simulink model "beamng_simulink_interface_demos"  (R2022b)
settings: Solver=FixedStepAuto  StartTime=0.0  StopTime=20  FixedStep=0.005  RelTol=1e-3
undefined symbols (not defined in the file): demo, mode
libraries: simulink x11, slpidlib x4, BeamNG_interface x1
settings Model: Creator=matti  LastModifiedBy=matti
settings SolverCC: AlgebraicLoopSolver=TrustRegion
settings DebuggingCC: ArithmeticOperatorsInVariantConditions=warning
settings SFSimCC: CustomCodeUndefinedFunction=UseInterfaceOnly

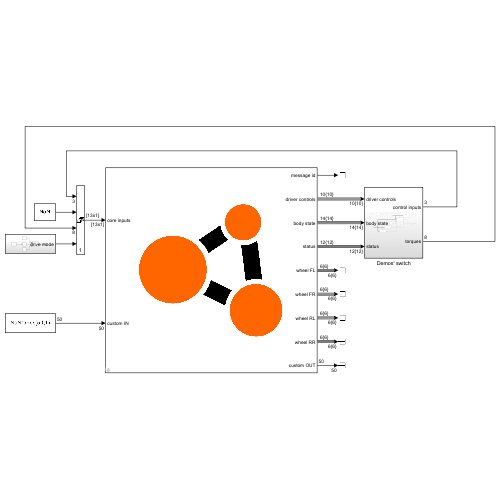
[thumbnail: Simulink's stored preview of the top-level diagram]
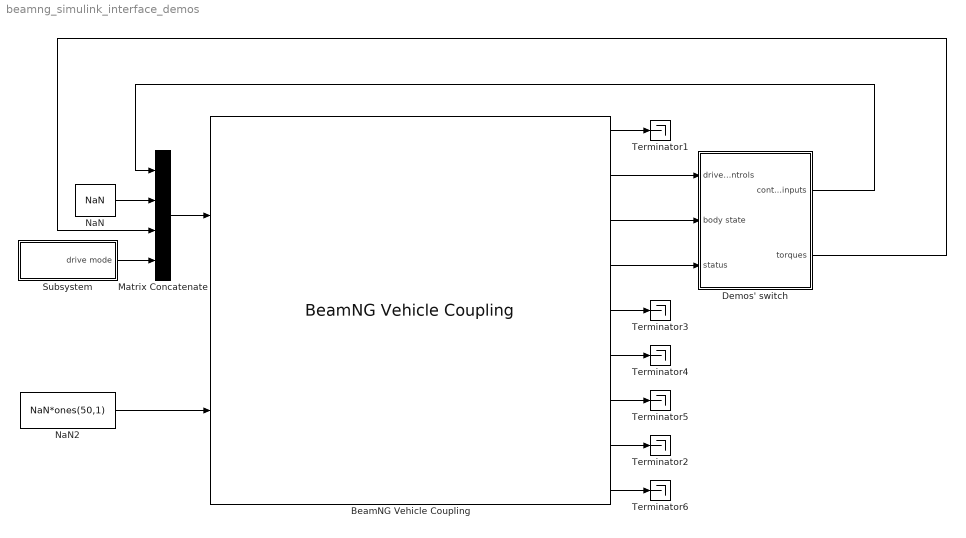
== system beamng_simulink_interface_demos ==
  BeamNG Vehicle Coupling : BeamNG_interface/BeamNG Vehicle Coupling
      settings: SourceProductName=BeamNG
  Demos' switch : Subsystem
  Matrix Concatenate : Concatenate  NumInputs=4  Mode=Multidimensional array
  NaN : Constant  Value=NaN  OutDataTypeStr=Inherit: Inherit via back propagation
  NaN2 : Constant  Value=NaN*ones(50,1)  OutDataTypeStr=Inherit: Inherit via back propagation
  Subsystem : Subsystem
  Terminator{1..6} (6 alike) : Terminator
  wires:
  Matrix Concatenate/1 -> BeamNG Vehicle Coupling/1
  NaN2/1 -> BeamNG Vehicle Coupling/2
  NaN/1 -> Matrix Concatenate/2
  BeamNG Vehicle Coupling/5 -> Terminator3/1
  BeamNG Vehicle Coupling/6 -> Terminator4/1
  BeamNG Vehicle Coupling/7 -> Terminator5/1
  BeamNG Vehicle Coupling/9 -> Terminator6/1
  Demos' switch/1(control inputs) -> Matrix Concatenate/1
  Demos' switch/2(torques) -> Matrix Concatenate/3
  Subsystem/1(drive mode) -> Matrix Concatenate/4
  BeamNG Vehicle Coupling/8 -> Terminator2/1
  BeamNG Vehicle Coupling/4 -> Demos' switch/3(status)
  BeamNG Vehicle Coupling/3 -> Demos' switch/2(body state)
  BeamNG Vehicle Coupling/2 -> Demos' switch/1(driver controls)
  BeamNG Vehicle Coupling/1 -> Terminator1/1

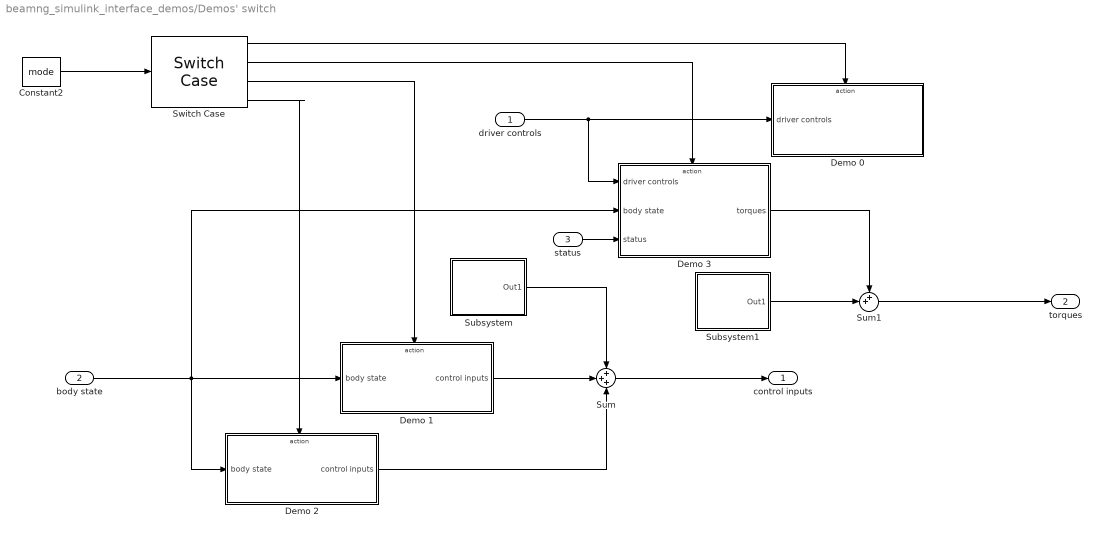
== system beamng_simulink_interface_demos/Demos' switch ==
  driver controls : Inport
  body state : Inport  Port=2
  status : Inport  Port=3
  Constant2 : Constant  Value=mode
  Demo 0 : Subsystem  TreatAsAtomicUnit=on
  Demo 1 : Subsystem  TreatAsAtomicUnit=on
  Demo 2 : Subsystem  TreatAsAtomicUnit=on
  Demo 3 : Subsystem  TreatAsAtomicUnit=on
  Subsystem : Subsystem
  Subsystem1 : Subsystem
  Sum : Sum  Inputs=+++
  Sum1 : Sum  Inputs=++|
  Switch Case : SwitchCase  CaseConditions={0, 3, 1, 2}  ShowDefaultCase=off
  control inputs : Outport
  torques : Outport  Port=2
  wires:
  Constant2/1 -> Switch Case/1
  Switch Case/1 -> Demo 0/Action
  Demo 2/1(control inputs) -> Sum/3
  driver controls/1 -> Demo 0/1(driver controls), Demo 3/1(driver controls)
  body state/1 -> Demo 3/2(body state), Demo 2/1(body state), Demo 1/1(body state)
  Sum/1 -> control inputs/1
  Subsystem/1(Out1) -> Sum/1
  Switch Case/4 -> Demo 2/Action
  Switch Case/3 -> Demo 1/Action
  Demo 1/1(control inputs) -> Sum/2
  Switch Case/2 -> Demo 3/Action
  Subsystem1/1(Out1) -> Sum1/2
  Demo 3/1(torques) -> Sum1/1
  Sum1/1 -> torques/1
  status/1 -> Demo 3/3(status)

== system beamng_simulink_interface_demos/Subsystem ==
  Compare To Constant : simulink/Logic and Bit Operations/Compare To Constant  relop===  const=3  OutDataTypeStr=boolean
  Constant : Constant  Value=mode
  Constant1 : Constant  Value=0
  Constant2 : Constant
  Switch : Switch  Criteria=u2 > Threshold  SaturateOnIntegerOverflow=off  InputSameDT=off
  drive mode : Outport
  wires:
  Constant/1 -> Compare To Constant/1
  Compare To Constant/1 -> Switch/2
  Constant1/1 -> Switch/3
  Constant2/1 -> Switch/1
  Switch/1 -> drive mode/1

== system beamng_simulink_interface_demos/Demos' switch/Demo 0 ==
  driver controls : Inport
  Action Port : ActionPort  ActionPortLabel=case [ 0 ]:
  Bus Selector : BusSelector  OutputSignals=throttle,brake,steering
  Scope : Scope  NumInputPorts=3
  To Workspace : ToWorkspace  VariableName=throttle0  SaveFormat=Timeseries  SampleTime=-1
  To Workspace1 : ToWorkspace  VariableName=brake0  SaveFormat=Timeseries  SampleTime=-1
  To Workspace2 : ToWorkspace  VariableName=steering0  SaveFormat=Timeseries  SampleTime=-1
  wires:
  driver controls/1 -> Bus Selector/1
  Bus Selector/1 -> To Workspace/1, Scope/1  "<throttle>"
  Bus Selector/2 -> To Workspace1/1, Scope/2  "<brake>"
  Bus Selector/3 -> To Workspace2/1, Scope/3  "<steering>"

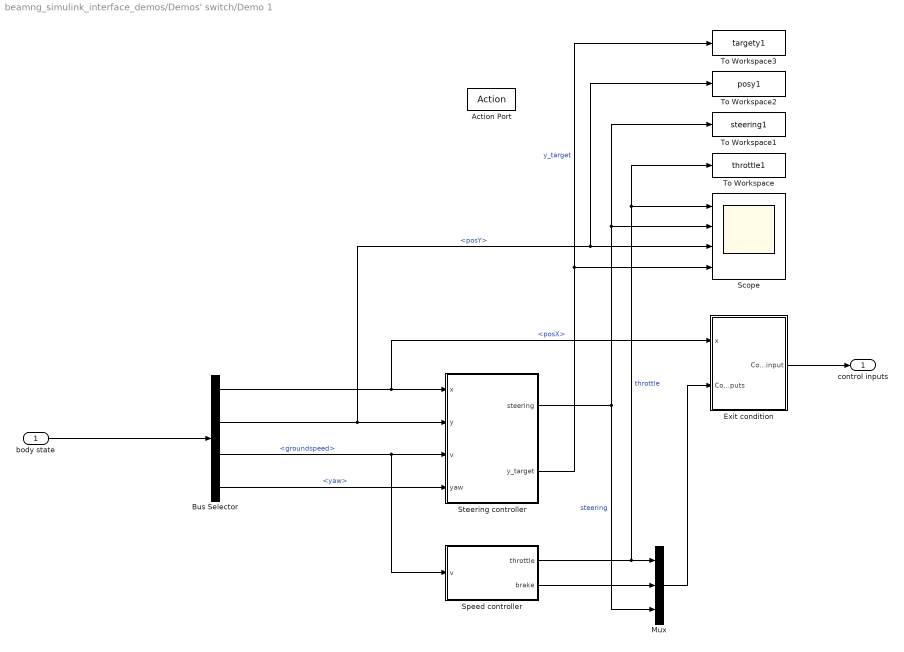
== system beamng_simulink_interface_demos/Demos' switch/Demo 1 ==
  body state : Inport
  Action Port : ActionPort  ActionPortLabel=case [ 1 ]:
  Bus Selector : BusSelector  OutputSignals=posX,posY,groundspeed,yaw
  Exit condition : Subsystem
  Mux : Mux  Inputs=3
  Scope : Scope  NumInputPorts=4
  Speed controller : Subsystem
  Steering controller : Subsystem
  To Workspace : ToWorkspace  VariableName=throttle1  SaveFormat=Timeseries  SampleTime=-1
  To Workspace1 : ToWorkspace  VariableName=steering1  SaveFormat=Timeseries  SampleTime=-1
  To Workspace2 : ToWorkspace  VariableName=posy1  SaveFormat=Timeseries  SampleTime=-1
  To Workspace3 : ToWorkspace  VariableName=targety1  SaveFormat=Timeseries  SampleTime=-1
  control inputs : Outport
  wires:
  Bus Selector/4 -> Steering controller/4(yaw)  "<yaw>"
  Speed controller/2(brake) -> Mux/2
  Exit condition/1(Control input) -> control inputs/1
  Mux/1 -> Exit condition/2(Control inputs)
  Speed controller/1(throttle) -> Mux/1, To Workspace/1, Scope/1  "throttle"
  body state/1 -> Bus Selector/1
  Bus Selector/2 -> Steering controller/2(y), To Workspace2/1, Scope/3  "<posY>"
  Bus Selector/1 -> Exit condition/1(x), Steering controller/1(x)  "<posX>"
  Steering controller/2(y_target) -> To Workspace3/1, Scope/4  "y_target"
  Bus Selector/3 -> Speed controller/1(v), Steering controller/3(v)  "<groundspeed>"
  Steering controller/1(steering) -> Mux/3, To Workspace1/1, Scope/2  "steering"

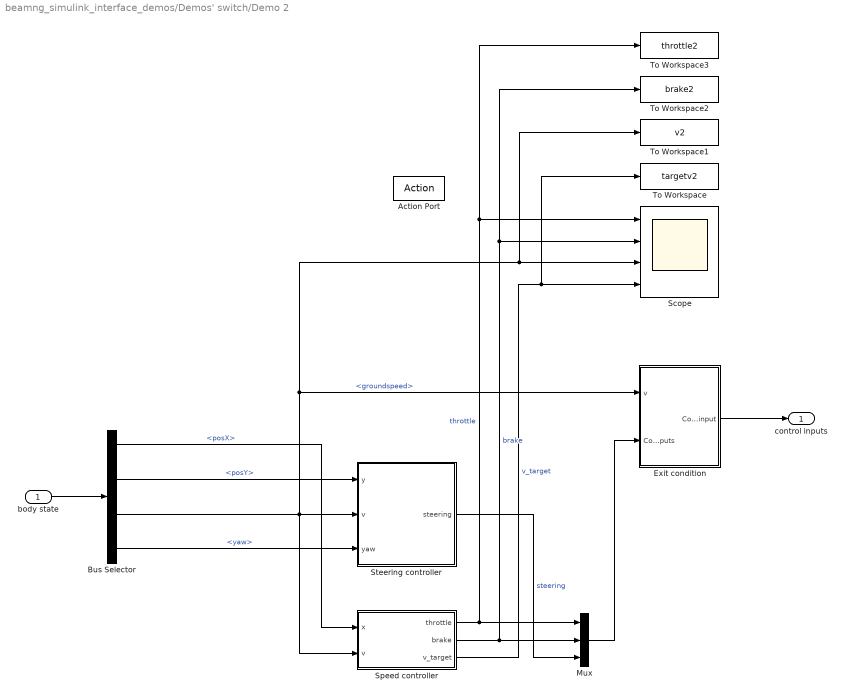
== system beamng_simulink_interface_demos/Demos' switch/Demo 2 ==
  body state : Inport
  Action Port : ActionPort  ActionPortLabel=case [ 2 ]:
  Bus Selector : BusSelector  OutputSignals=posX,posY,groundspeed,yaw
  Exit condition : Subsystem
  Mux : Mux  Inputs=3
  Scope : Scope  NumInputPorts=4
  Speed controller : Subsystem
  Steering controller : Subsystem
  To Workspace : ToWorkspace  VariableName=targetv2  SaveFormat=Timeseries  SampleTime=-1
  To Workspace1 : ToWorkspace  VariableName=v2  SaveFormat=Timeseries  SampleTime=-1
  To Workspace2 : ToWorkspace  VariableName=brake2  SaveFormat=Timeseries  SampleTime=-1
  To Workspace3 : ToWorkspace  VariableName=throttle2  SaveFormat=Timeseries  SampleTime=-1
  control inputs : Outport
  wires:
  Speed controller/3(v_target) -> To Workspace/1, Scope/4  "v_target"
  Exit condition/1(Control input) -> control inputs/1
  Speed controller/2(brake) -> Mux/2, To Workspace2/1, Scope/2  "brake"
  Steering controller/1(steering) -> Mux/3  "steering"
  Speed controller/1(throttle) -> Mux/1, To Workspace3/1, Scope/1  "throttle"
  body state/1 -> Bus Selector/1
  Bus Selector/4 -> Steering controller/3(yaw)  "<yaw>"
  Mux/1 -> Exit condition/2(Control inputs)
  Bus Selector/3 -> Speed controller/2(v), To Workspace1/1, Scope/3, Exit condition/1(v), Steering controller/2(v)  "<groundspeed>"
  Bus Selector/2 -> Steering controller/1(y)  "<posY>"
  Bus Selector/1 -> Speed controller/1(x)  "<posX>"

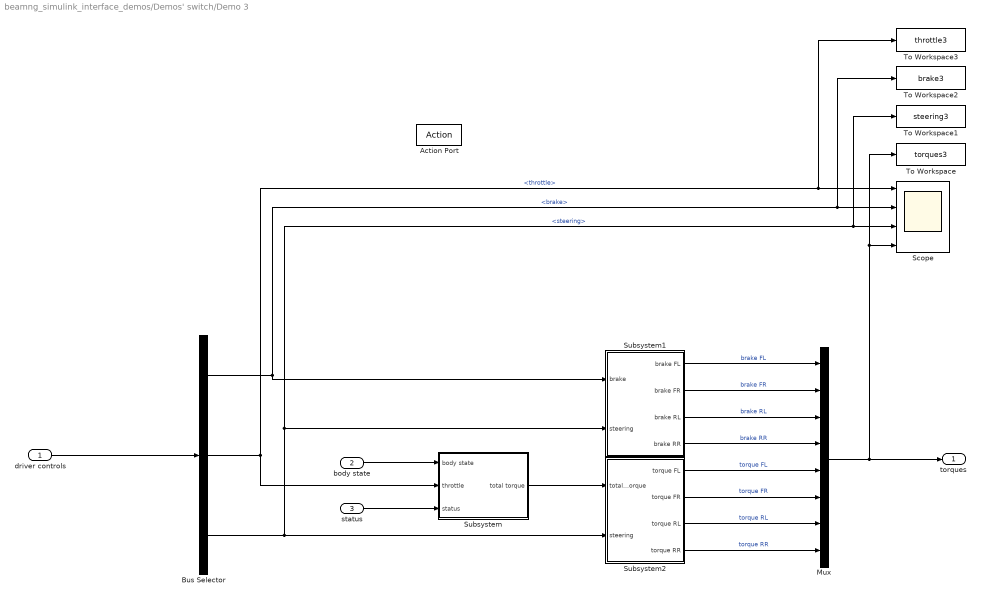
== system beamng_simulink_interface_demos/Demos' switch/Demo 3 ==
  driver controls : Inport
  body state : Inport  Port=2
  status : Inport  Port=3
  Action Port : ActionPort  ActionPortLabel=case [ 3 ]:
  Bus Selector : BusSelector  OutputSignals=brake,throttle,steering
  Mux : Mux  Inputs=8
  Scope : Scope  NumInputPorts=4
  Subsystem : Subsystem
  Subsystem1 : Subsystem
  Subsystem2 : Subsystem
  To Workspace : ToWorkspace  VariableName=torques3  SaveFormat=Timeseries  SampleTime=-1
  To Workspace1 : ToWorkspace  VariableName=steering3  SaveFormat=Timeseries  SampleTime=-1
  To Workspace2 : ToWorkspace  VariableName=brake3  SaveFormat=Timeseries  SampleTime=-1
  To Workspace3 : ToWorkspace  VariableName=throttle3  SaveFormat=Timeseries  SampleTime=-1
  torques : Outport
  wires:
  driver controls/1 -> Bus Selector/1
  Bus Selector/1 -> Subsystem1/1(brake), To Workspace2/1, Scope/2  "<brake>"
  Bus Selector/2 -> Subsystem/2(throttle), To Workspace3/1, Scope/1  "<throttle>"
  Bus Selector/3 -> Subsystem1/2(steering), To Workspace1/1, Scope/3, Subsystem2/2(steering)  "<steering>"
  body state/1 -> Subsystem/1(body state)
  status/1 -> Subsystem/3(status)
  Subsystem1/1(brake FL) -> Mux/1  "brake FL"
  Subsystem1/2(brake FR) -> Mux/2  "brake FR"
  Subsystem1/3(brake RL) -> Mux/3  "brake RL"
  Subsystem1/4(brake RR) -> Mux/4  "brake RR"
  Subsystem/1(total torque) -> Subsystem2/1(total torque)
  Subsystem2/1(torque FL) -> Mux/5  "torque FL"
  Subsystem2/2(torque FR) -> Mux/6  "torque FR"
  Subsystem2/3(torque RL) -> Mux/7  "torque RL"
  Subsystem2/4(torque RR) -> Mux/8  "torque RR"
  Mux/1 -> torques/1, To Workspace/1, Scope/4

== system beamng_simulink_interface_demos/Demos' switch/Subsystem ==
  Compare To Constant : simulink/Logic and Bit Operations/Compare To Constant  relop===  const=0  OutDataTypeStr=boolean
  Compare To Constant1 : simulink/Logic and Bit Operations/Compare To Constant  relop===  const=3  OutDataTypeStr=boolean
  Constant : Constant  Value=mode
  NaN : Constant  Value=NaN*ones(3,1)  OutDataTypeStr=Inherit: Inherit via back propagation
  NaN2 : Constant  Value=zeros(3,1)  OutDataTypeStr=Inherit: Inherit via back propagation
  OR : Logic  Operator=OR  IconShape=distinctive  AllPortsSameDT=off  OutDataTypeStr=boolean
  Switch : Switch  Criteria=u2 > Threshold  SaturateOnIntegerOverflow=off  InputSameDT=off
  Out1 : Outport
  wires:
  Constant/1 -> Compare To Constant1/1, Compare To Constant/1
  NaN/1 -> Switch/1
  Compare To Constant/1 -> OR/1
  OR/1 -> Switch/2
  NaN2/1 -> Switch/3
  Switch/1 -> Out1/1
  Compare To Constant1/1 -> OR/2

== system beamng_simulink_interface_demos/Demos' switch/Subsystem1 ==
  Compare To Constant1 : simulink/Logic and Bit Operations/Compare To Constant  relop===  const=3  OutDataTypeStr=boolean
  Constant : Constant  Value=mode
  NaN : Constant  Value=NaN*ones(8,1)  OutDataTypeStr=Inherit: Inherit via back propagation
  NaN2 : Constant  Value=zeros(8,1)  OutDataTypeStr=Inherit: Inherit via back propagation
  Switch : Switch  Criteria=u2 > Threshold  SaturateOnIntegerOverflow=off  InputSameDT=off
  Out1 : Outport
  wires:
  Switch/1 -> Out1/1
  Compare To Constant1/1 -> Switch/2
  Constant/1 -> Compare To Constant1/1
  NaN2/1 -> Switch/1
  NaN/1 -> Switch/3

== system beamng_simulink_interface_demos/Demos' switch/Demo 1/Exit condition ==
  x : Inport
  Control inputs : Inport  Port=2
  Constant3 : Constant
  Stop Simulation : Stop
  Switch1 : Switch  Threshold=demo(1).x4  SaturateOnIntegerOverflow=off  InputSameDT=off
  Switch2 : Switch  Criteria=u2 > Threshold  Threshold=demo(1).x4  SaturateOnIntegerOverflow=off  InputSameDT=off
  Zero : Constant  Value=0  OutDataTypeStr=Inherit: Inherit via back propagation
  Zero1 : Constant  Value=zeros(3,1)  OutDataTypeStr=Inherit: Inherit via back propagation
  Control input : Outport
  wires:
  Zero/1 -> Switch2/3
  x/1 -> Switch1/2, Switch2/2
  Switch2/1 -> Stop Simulation/1
  Constant3/1 -> Switch2/1
  Control inputs/1 -> Switch1/3
  Switch1/1 -> Control input/1
  Zero1/1 -> Switch1/1

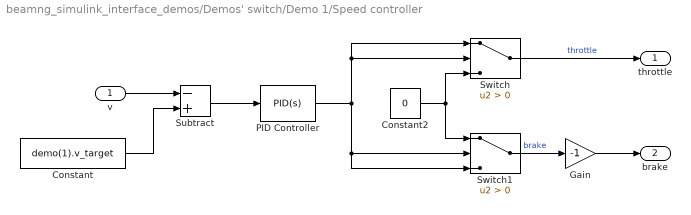
== system beamng_simulink_interface_demos/Demos' switch/Demo 1/Speed controller ==
  v : Inport
  Constant : Constant  Value=demo(1).v_target
  Constant2 : Constant  Value=0
  Gain : Gain  Gain=-1
  PID Controller : slpidlib/PID Controller  Controller=PID  Form=Parallel  TimeDomain=Continuous-time  UseExternalTs=off  SampleTime=-1  IntegratorMethod=Forward Euler  FilterMethod=Forward Euler  ControllerParametersSource=internal  P=0.1  I=0.01  UseKiTs=off  D=0  N=100  UseFilter=on  TunerSelectOption=Transfer Function Based (PID Tuner App)  InitialConditionSource=internal  InitialConditionForIntegrator=0  InitialConditionForFilter=0  DifferentiatorICPrevScaledInput=0  ExternalReset=none  TrackingMode=off  Kt=1  LimitOutput=on  SatLimitsSource=internal  UpperSaturationLimit=1  LowerSaturationLimit=-1  LinearizeAsGain=on  AntiWindupMode=none  Kb=1  LimitIntegrator=off  UpperIntegratorSaturationLimit=inf  LowerIntegratorSaturationLimit=-inf  POutMin=[]  POutMax=[]  IOutMin=[]  IOutMax=[]  DOutMin=[]  DOutMax=[]  NOutMin=[]  NOutMax=[]  SumOutMin=[]  SumOutMax=[]  SaturationOutMin=[]  SaturationOutMax=[]  PParamMin=[]  PParamMax=[]  IParamMin=[]  IParamMax=[]  DParamMin=[]  DParamMax=[]  NParamMin=[]  NParamMax=[]  KbParamMin=[]  KbParamMax=[]  KtParamMin=[]  KtParamMax=[]  KbOutMin=[]  KbOutMax=[]  KtOutMin=[]  KtOutMax=[]  IntegratorOutMin=[]  IntegratorOutMax=[]  FilterOutMin=[]  FilterOutMax=[]  SumI1OutMin=[]  SumI1OutMax=[]  SumI2OutMin=[]  SumI2OutMax=[]  SumI3OutMin=[]  SumI3OutMax=[]  SumI4OutMin=[]  SumI4OutMax=[]  SumDOutMin=[]  SumDOutMax=[]  DifferentiatorOutMin=[]  DifferentiatorOutMax=[]  FilterDiffOutCoefMin=[]  FilterDiffOutCoefMax=[]  ReciprocalOutMin=[]  ReciprocalOutMax=[]  SumDenOutMin=[]  SumDenOutMax=[]  SumNumOutMin=[]  SumNumOutMax=[]  DivideOutMin=[]  DivideOutMax=[]  UdiffTsProdOutMin=[]  UdiffTsProdOutMax=[]  NTsProdOutMin=[]  NTsProdOutMax=[]  UintegralTsProdOutMin=[]  UintegralTsProdOutMax=[]  UngainTsProdOutMin=[]  UngainTsProdOutMax=[]  ClampingZeroOutDataTypeStr=Inherit: Inherit via back propagation  ClampingZeroOutMin=[]  ClampingZeroOutMax=[]  FilterDenConstantOutDataTypeStr=Inherit: Inherit via back propagation  FilterDenConstantOutMin=[]  FilterDenConstantOutMax=[]  PCopyOutDataTypeStr=Inherit: Inherit via back propagation  PCopyOutMin=[]  PCopyOutMax=[]  NCopyOutDataTypeStr=Inherit: Inherit via back propagation  NCopyOutMin=[]  NCopyOutMax=[]  IntegratorContinuousStateAttributes=''  IntegratorStateMustResolveToSignalObject=off  IntegratorRTWStateStorageClass=Auto  FilterContinuousStateAttributes=''  FilterStateMustResolveToSignalObject=off  FilterRTWStateStorageClass=Auto  ParallelPVariant=InternalParameters  IdealPVariant=Disabled  IVariant=InternalParameters  DVariant=InternalParameters  IntegratorVariant=Continuous  SatVariant=Enabled  AWVariant=Passthrough  PCopyVariant=Disabled  TRVariant=Disabled  FdbkBlocksVariant=Forward  IdealPFdbkVariant=Disabled  SatFdbkVariant=Disabled  DerivativeFilterVariant=ContFilter  NVariant=InternalParameters  NCopyVariant=Disabled  FilterICVariant=InternalICsFilter  IntegratorICVariant=InternalICs  ExternalResetVariant=Disabled  TRSumVariant=Passthrough  SumFdbkVariant=Disabled  SumVariant=Sum_PID  TsampFilterVariant=InternalTs  TsampNgainVariant=Passthrough  TsampIntegralVariant=Passthrough  ExternalSaturationOutDataTypeStr=Inherit: Same as second input
  Subtract : Sum  Inputs=-+
  Switch : Switch  Criteria=u2 > Threshold  SaturateOnIntegerOverflow=off  InputSameDT=off
  Switch1 : Switch  Criteria=u2 > Threshold  SaturateOnIntegerOverflow=off  InputSameDT=off
  throttle : Outport
  brake : Outport  Port=2
  wires:
  PID Controller/1 -> Switch/2, Switch/1, Switch1/2, Switch1/3
  v/1 -> Subtract/1
  Constant2/1 -> Switch/3, Switch1/1
  Switch1/1 -> Gain/1  "brake"
  Constant/1 -> Subtract/2
  Subtract/1 -> PID Controller/1
  Switch/1 -> throttle/1  "throttle"
  Gain/1 -> brake/1

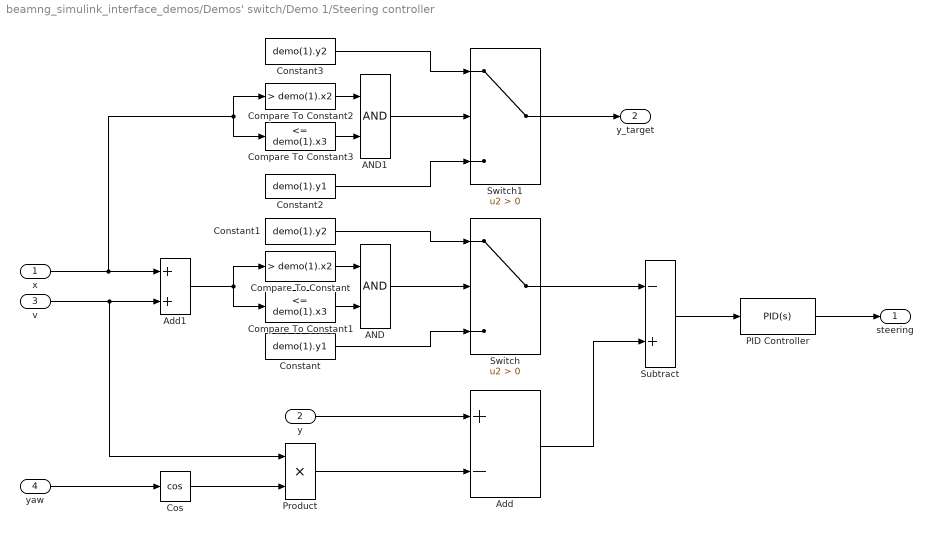
== system beamng_simulink_interface_demos/Demos' switch/Demo 1/Steering controller ==
  x : Inport
  y : Inport  Port=2
  v : Inport  Port=3
  yaw : Inport  Port=4
  AND : Logic  IconShape=distinctive  AllPortsSameDT=off  OutDataTypeStr=boolean
  AND1 : Logic  IconShape=distinctive  AllPortsSameDT=off  OutDataTypeStr=boolean
  Add : Sum  Inputs=+-
  Add1 : Sum
  Compare To Constant : simulink/Logic and Bit Operations/Compare To Constant  relop=>  const=demo(1).x2  OutDataTypeStr=boolean
  Compare To Constant1 : simulink/Logic and Bit Operations/Compare To Constant  relop=<=  const=demo(1).x3  OutDataTypeStr=boolean
  Compare To Constant2 : simulink/Logic and Bit Operations/Compare To Constant  relop=>  const=demo(1).x2  OutDataTypeStr=boolean
  Compare To Constant3 : simulink/Logic and Bit Operations/Compare To Constant  relop=<=  const=demo(1).x3  OutDataTypeStr=boolean
  Constant : Constant  Value=demo(1).y1
  Constant1 : Constant  Value=demo(1).y2
  Constant2 : Constant  Value=demo(1).y1
  Constant3 : Constant  Value=demo(1).y2
  Cos : Trigonometry  Operator=cos
  PID Controller : slpidlib/PID Controller  Controller=PID  Form=Parallel  TimeDomain=Continuous-time  UseExternalTs=off  SampleTime=-1  IntegratorMethod=Forward Euler  FilterMethod=Forward Euler  ControllerParametersSource=internal  P=0.05  I=0  UseKiTs=off  D=0  N=100  UseFilter=on  TunerSelectOption=Transfer Function Based (PID Tuner App)  InitialConditionSource=internal  InitialConditionForIntegrator=0  InitialConditionForFilter=0  DifferentiatorICPrevScaledInput=0  ExternalReset=none  TrackingMode=off  Kt=1  LimitOutput=on  SatLimitsSource=internal  UpperSaturationLimit=1  LowerSaturationLimit=-1  LinearizeAsGain=on  AntiWindupMode=none  Kb=1  LimitIntegrator=off  UpperIntegratorSaturationLimit=inf  LowerIntegratorSaturationLimit=-inf  POutMin=[]  POutMax=[]  IOutMin=[]  IOutMax=[]  DOutMin=[]  DOutMax=[]  NOutMin=[]  NOutMax=[]  SumOutMin=[]  SumOutMax=[]  SaturationOutMin=[]  SaturationOutMax=[]  PParamMin=[]  PParamMax=[]  IParamMin=[]  IParamMax=[]  DParamMin=[]  DParamMax=[]  NParamMin=[]  NParamMax=[]  KbParamMin=[]  KbParamMax=[]  KtParamMin=[]  KtParamMax=[]  KbOutMin=[]  KbOutMax=[]  KtOutMin=[]  KtOutMax=[]  IntegratorOutMin=[]  IntegratorOutMax=[]  FilterOutMin=[]  FilterOutMax=[]  SumI1OutMin=[]  SumI1OutMax=[]  SumI2OutMin=[]  SumI2OutMax=[]  SumI3OutMin=[]  SumI3OutMax=[]  SumI4OutMin=[]  SumI4OutMax=[]  SumDOutMin=[]  SumDOutMax=[]  DifferentiatorOutMin=[]  DifferentiatorOutMax=[]  FilterDiffOutCoefMin=[]  FilterDiffOutCoefMax=[]  ReciprocalOutMin=[]  ReciprocalOutMax=[]  SumDenOutMin=[]  SumDenOutMax=[]  SumNumOutMin=[]  SumNumOutMax=[]  DivideOutMin=[]  DivideOutMax=[]  UdiffTsProdOutMin=[]  UdiffTsProdOutMax=[]  NTsProdOutMin=[]  NTsProdOutMax=[]  UintegralTsProdOutMin=[]  UintegralTsProdOutMax=[]  UngainTsProdOutMin=[]  UngainTsProdOutMax=[]  ClampingZeroOutDataTypeStr=Inherit: Inherit via back propagation  ClampingZeroOutMin=[]  ClampingZeroOutMax=[]  FilterDenConstantOutDataTypeStr=Inherit: Inherit via back propagation  FilterDenConstantOutMin=[]  FilterDenConstantOutMax=[]  PCopyOutDataTypeStr=Inherit: Inherit via back propagation  PCopyOutMin=[]  PCopyOutMax=[]  NCopyOutDataTypeStr=Inherit: Inherit via back propagation  NCopyOutMin=[]  NCopyOutMax=[]  IntegratorContinuousStateAttributes=''  IntegratorStateMustResolveToSignalObject=off  IntegratorRTWStateStorageClass=Auto  FilterContinuousStateAttributes=''  FilterStateMustResolveToSignalObject=off  FilterRTWStateStorageClass=Auto  ParallelPVariant=InternalParameters  IdealPVariant=Disabled  IVariant=InternalParameters  DVariant=InternalParameters  IntegratorVariant=Continuous  SatVariant=Enabled  AWVariant=Passthrough  PCopyVariant=Disabled  TRVariant=Disabled  FdbkBlocksVariant=Forward  IdealPFdbkVariant=Disabled  SatFdbkVariant=Disabled  DerivativeFilterVariant=ContFilter  NVariant=InternalParameters  NCopyVariant=Disabled  FilterICVariant=InternalICsFilter  IntegratorICVariant=InternalICs  ExternalResetVariant=Disabled  TRSumVariant=Passthrough  SumFdbkVariant=Disabled  SumVariant=Sum_PID  TsampFilterVariant=InternalTs  TsampNgainVariant=Passthrough  TsampIntegralVariant=Passthrough  ExternalSaturationOutDataTypeStr=Inherit: Same as second input
  Product : Product
  Subtract : Sum  Inputs=-+
  Switch : Switch  Criteria=u2 > Threshold  SaturateOnIntegerOverflow=off  InputSameDT=off
  Switch1 : Switch  Criteria=u2 > Threshold  SaturateOnIntegerOverflow=off  InputSameDT=off
  steering : Outport
  y_target : Outport  Port=2
  wires:
  v/1 -> Product/1, Add1/2
  Add1/1 -> Compare To Constant/1, Compare To Constant1/1
  Compare To Constant/1 -> AND/1
  Compare To Constant1/1 -> AND/2
  AND/1 -> Switch/2
  Constant1/1 -> Switch/1
  Constant/1 -> Switch/3
  Switch/1 -> Subtract/1
  PID Controller/1 -> steering/1
  Subtract/1 -> PID Controller/1
  yaw/1 -> Cos/1
  Cos/1 -> Product/2
  Product/1 -> Add/2
  y/1 -> Add/1
  Add/1 -> Subtract/2
  Switch1/1 -> y_target/1
  Constant2/1 -> Switch1/3
  Constant3/1 -> Switch1/1
  AND1/1 -> Switch1/2
  Compare To Constant3/1 -> AND1/2
  Compare To Constant2/1 -> AND1/1
  x/1 -> Compare To Constant2/1, Compare To Constant3/1, Add1/1

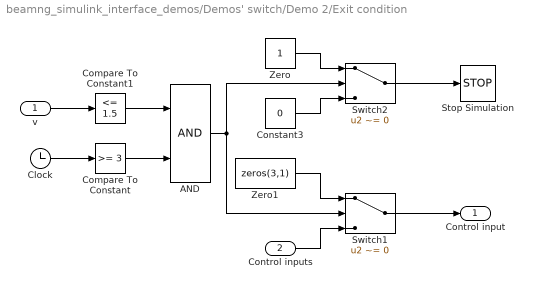
== system beamng_simulink_interface_demos/Demos' switch/Demo 2/Exit condition ==
  v : Inport
  Control inputs : Inport  Port=2
  AND : Logic  IconShape=distinctive  AllPortsSameDT=off  OutDataTypeStr=boolean
  Clock : Clock
  Compare To Constant : simulink/Logic and Bit Operations/Compare To Constant  relop=>=  const=3  OutDataTypeStr=boolean
  Compare To Constant1 : simulink/Logic and Bit Operations/Compare To Constant  relop=<=  const=1.5  OutDataTypeStr=boolean
  Constant3 : Constant  Value=0
  Stop Simulation : Stop
  Switch1 : Switch  Criteria=u2 ~= 0  SaturateOnIntegerOverflow=off  InputSameDT=off
  Switch2 : Switch  Criteria=u2 ~= 0  SaturateOnIntegerOverflow=off  InputSameDT=off
  Zero : Constant  OutDataTypeStr=Inherit: Inherit via back propagation
  Zero1 : Constant  Value=zeros(3,1)  OutDataTypeStr=Inherit: Inherit via back propagation
  Control input : Outport
  wires:
  Switch2/1 -> Stop Simulation/1
  Switch1/1 -> Control input/1
  Clock/1 -> Compare To Constant/1
  v/1 -> Compare To Constant1/1
  Compare To Constant1/1 -> AND/1
  Compare To Constant/1 -> AND/2
  Constant3/1 -> Switch2/3
  Zero/1 -> Switch2/1
  AND/1 -> Switch1/2, Switch2/2
  Zero1/1 -> Switch1/1
  Control inputs/1 -> Switch1/3

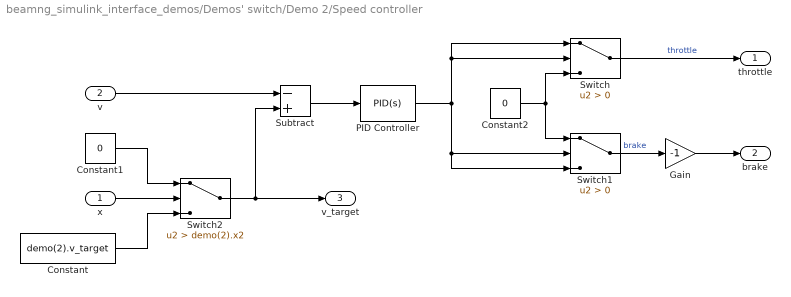
== system beamng_simulink_interface_demos/Demos' switch/Demo 2/Speed controller ==
  x : Inport
  v : Inport  Port=2
  Constant : Constant  Value=demo(2).v_target
  Constant1 : Constant  Value=0
  Constant2 : Constant  Value=0
  Gain : Gain  Gain=-1
  PID Controller : slpidlib/PID Controller  Controller=PID  Form=Parallel  TimeDomain=Continuous-time  UseExternalTs=off  SampleTime=-1  IntegratorMethod=Forward Euler  FilterMethod=Forward Euler  ControllerParametersSource=internal  P=0.3  I=0.001  UseKiTs=off  D=0  N=100  UseFilter=on  TunerSelectOption=Transfer Function Based (PID Tuner App)  InitialConditionSource=internal  InitialConditionForIntegrator=0  InitialConditionForFilter=0  DifferentiatorICPrevScaledInput=0  ExternalReset=none  TrackingMode=off  Kt=1  LimitOutput=on  SatLimitsSource=internal  UpperSaturationLimit=1  LowerSaturationLimit=-1  LinearizeAsGain=on  AntiWindupMode=none  Kb=1  LimitIntegrator=off  UpperIntegratorSaturationLimit=inf  LowerIntegratorSaturationLimit=-inf  POutMin=[]  POutMax=[]  IOutMin=[]  IOutMax=[]  DOutMin=[]  DOutMax=[]  NOutMin=[]  NOutMax=[]  SumOutMin=[]  SumOutMax=[]  SaturationOutMin=[]  SaturationOutMax=[]  PParamMin=[]  PParamMax=[]  IParamMin=[]  IParamMax=[]  DParamMin=[]  DParamMax=[]  NParamMin=[]  NParamMax=[]  KbParamMin=[]  KbParamMax=[]  KtParamMin=[]  KtParamMax=[]  KbOutMin=[]  KbOutMax=[]  KtOutMin=[]  KtOutMax=[]  IntegratorOutMin=[]  IntegratorOutMax=[]  FilterOutMin=[]  FilterOutMax=[]  SumI1OutMin=[]  SumI1OutMax=[]  SumI2OutMin=[]  SumI2OutMax=[]  SumI3OutMin=[]  SumI3OutMax=[]  SumI4OutMin=[]  SumI4OutMax=[]  SumDOutMin=[]  SumDOutMax=[]  DifferentiatorOutMin=[]  DifferentiatorOutMax=[]  FilterDiffOutCoefMin=[]  FilterDiffOutCoefMax=[]  ReciprocalOutMin=[]  ReciprocalOutMax=[]  SumDenOutMin=[]  SumDenOutMax=[]  SumNumOutMin=[]  SumNumOutMax=[]  DivideOutMin=[]  DivideOutMax=[]  UdiffTsProdOutMin=[]  UdiffTsProdOutMax=[]  NTsProdOutMin=[]  NTsProdOutMax=[]  UintegralTsProdOutMin=[]  UintegralTsProdOutMax=[]  UngainTsProdOutMin=[]  UngainTsProdOutMax=[]  ClampingZeroOutDataTypeStr=Inherit: Inherit via back propagation  ClampingZeroOutMin=[]  ClampingZeroOutMax=[]  FilterDenConstantOutDataTypeStr=Inherit: Inherit via back propagation  FilterDenConstantOutMin=[]  FilterDenConstantOutMax=[]  PCopyOutDataTypeStr=Inherit: Inherit via back propagation  PCopyOutMin=[]  PCopyOutMax=[]  NCopyOutDataTypeStr=Inherit: Inherit via back propagation  NCopyOutMin=[]  NCopyOutMax=[]  IntegratorContinuousStateAttributes=''  IntegratorStateMustResolveToSignalObject=off  IntegratorRTWStateStorageClass=Auto  FilterContinuousStateAttributes=''  FilterStateMustResolveToSignalObject=off  FilterRTWStateStorageClass=Auto  ParallelPVariant=InternalParameters  IdealPVariant=Disabled  IVariant=InternalParameters  DVariant=InternalParameters  IntegratorVariant=Continuous  SatVariant=Enabled  AWVariant=Passthrough  PCopyVariant=Disabled  TRVariant=Disabled  FdbkBlocksVariant=Forward  IdealPFdbkVariant=Disabled  SatFdbkVariant=Disabled  DerivativeFilterVariant=ContFilter  NVariant=InternalParameters  NCopyVariant=Disabled  FilterICVariant=InternalICsFilter  IntegratorICVariant=InternalICs  ExternalResetVariant=Disabled  TRSumVariant=Passthrough  SumFdbkVariant=Disabled  SumVariant=Sum_PID  TsampFilterVariant=InternalTs  TsampNgainVariant=Passthrough  TsampIntegralVariant=Passthrough  ExternalSaturationOutDataTypeStr=Inherit: Same as second input
  Subtract : Sum  Inputs=-+
  Switch : Switch  Criteria=u2 > Threshold  SaturateOnIntegerOverflow=off  InputSameDT=off
  Switch1 : Switch  Criteria=u2 > Threshold  SaturateOnIntegerOverflow=off  InputSameDT=off
  Switch2 : Switch  Criteria=u2 > Threshold  Threshold=demo(2).x2  SaturateOnIntegerOverflow=off  InputSameDT=off
  throttle : Outport
  brake : Outport  Port=2
  v_target : Outport  Port=3
  wires:
  PID Controller/1 -> Switch/2, Switch/1, Switch1/2, Switch1/3
  v/1 -> Subtract/1
  Constant2/1 -> Switch/3, Switch1/1
  Switch1/1 -> Gain/1  "brake"
  Subtract/1 -> PID Controller/1
  Switch/1 -> throttle/1  "throttle"
  x/1 -> Switch2/2
  Switch2/1 -> v_target/1, Subtract/2
  Gain/1 -> brake/1
  Constant1/1 -> Switch2/1
  Constant/1 -> Switch2/3

== system beamng_simulink_interface_demos/Demos' switch/Demo 2/Steering controller ==
  y : Inport
  v : Inport  Port=2
  yaw : Inport  Port=3
  Add : Sum  Inputs=+-
  Constant : Constant  Value=demo(2).y
  Cos : Trigonometry  Operator=cos
  PID Controller : slpidlib/PID Controller  Controller=PID  Form=Parallel  TimeDomain=Continuous-time  UseExternalTs=off  SampleTime=-1  IntegratorMethod=Forward Euler  FilterMethod=Forward Euler  ControllerParametersSource=internal  P=0.05  I=0  UseKiTs=off  D=0  N=100  UseFilter=on  TunerSelectOption=Transfer Function Based (PID Tuner App)  InitialConditionSource=internal  InitialConditionForIntegrator=0  InitialConditionForFilter=0  DifferentiatorICPrevScaledInput=0  ExternalReset=none  TrackingMode=off  Kt=1  LimitOutput=on  SatLimitsSource=internal  UpperSaturationLimit=1  LowerSaturationLimit=-1  LinearizeAsGain=on  AntiWindupMode=none  Kb=1  LimitIntegrator=off  UpperIntegratorSaturationLimit=inf  LowerIntegratorSaturationLimit=-inf  POutMin=[]  POutMax=[]  IOutMin=[]  IOutMax=[]  DOutMin=[]  DOutMax=[]  NOutMin=[]  NOutMax=[]  SumOutMin=[]  SumOutMax=[]  SaturationOutMin=[]  SaturationOutMax=[]  PParamMin=[]  PParamMax=[]  IParamMin=[]  IParamMax=[]  DParamMin=[]  DParamMax=[]  NParamMin=[]  NParamMax=[]  KbParamMin=[]  KbParamMax=[]  KtParamMin=[]  KtParamMax=[]  KbOutMin=[]  KbOutMax=[]  KtOutMin=[]  KtOutMax=[]  IntegratorOutMin=[]  IntegratorOutMax=[]  FilterOutMin=[]  FilterOutMax=[]  SumI1OutMin=[]  SumI1OutMax=[]  SumI2OutMin=[]  SumI2OutMax=[]  SumI3OutMin=[]  SumI3OutMax=[]  SumI4OutMin=[]  SumI4OutMax=[]  SumDOutMin=[]  SumDOutMax=[]  DifferentiatorOutMin=[]  DifferentiatorOutMax=[]  FilterDiffOutCoefMin=[]  FilterDiffOutCoefMax=[]  ReciprocalOutMin=[]  ReciprocalOutMax=[]  SumDenOutMin=[]  SumDenOutMax=[]  SumNumOutMin=[]  SumNumOutMax=[]  DivideOutMin=[]  DivideOutMax=[]  UdiffTsProdOutMin=[]  UdiffTsProdOutMax=[]  NTsProdOutMin=[]  NTsProdOutMax=[]  UintegralTsProdOutMin=[]  UintegralTsProdOutMax=[]  UngainTsProdOutMin=[]  UngainTsProdOutMax=[]  ClampingZeroOutDataTypeStr=Inherit: Inherit via back propagation  ClampingZeroOutMin=[]  ClampingZeroOutMax=[]  FilterDenConstantOutDataTypeStr=Inherit: Inherit via back propagation  FilterDenConstantOutMin=[]  FilterDenConstantOutMax=[]  PCopyOutDataTypeStr=Inherit: Inherit via back propagation  PCopyOutMin=[]  PCopyOutMax=[]  NCopyOutDataTypeStr=Inherit: Inherit via back propagation  NCopyOutMin=[]  NCopyOutMax=[]  IntegratorContinuousStateAttributes=''  IntegratorStateMustResolveToSignalObject=off  IntegratorRTWStateStorageClass=Auto  FilterContinuousStateAttributes=''  FilterStateMustResolveToSignalObject=off  FilterRTWStateStorageClass=Auto  ParallelPVariant=InternalParameters  IdealPVariant=Disabled  IVariant=InternalParameters  DVariant=InternalParameters  IntegratorVariant=Continuous  SatVariant=Enabled  AWVariant=Passthrough  PCopyVariant=Disabled  TRVariant=Disabled  FdbkBlocksVariant=Forward  IdealPFdbkVariant=Disabled  SatFdbkVariant=Disabled  DerivativeFilterVariant=ContFilter  NVariant=InternalParameters  NCopyVariant=Disabled  FilterICVariant=InternalICsFilter  IntegratorICVariant=InternalICs  ExternalResetVariant=Disabled  TRSumVariant=Passthrough  SumFdbkVariant=Disabled  SumVariant=Sum_PID  TsampFilterVariant=InternalTs  TsampNgainVariant=Passthrough  TsampIntegralVariant=Passthrough  ExternalSaturationOutDataTypeStr=Inherit: Same as second input
  Product : Product
  Subtract : Sum  Inputs=-+
  steering : Outport
  wires:
  v/1 -> Product/1
  Constant/1 -> Subtract/1
  PID Controller/1 -> steering/1
  Subtract/1 -> PID Controller/1
  yaw/1 -> Cos/1
  Cos/1 -> Product/2
  Product/1 -> Add/2
  y/1 -> Add/1
  Add/1 -> Subtract/2

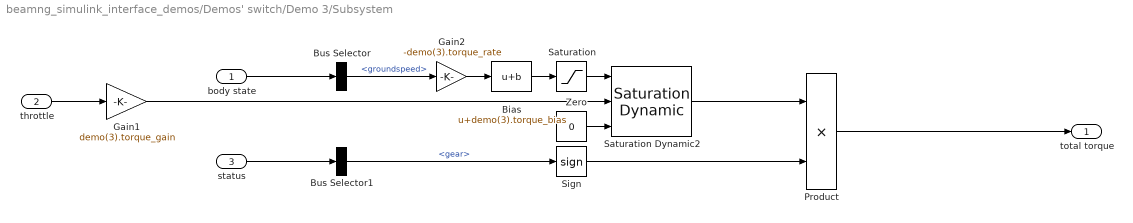
== system beamng_simulink_interface_demos/Demos' switch/Demo 3/Subsystem ==
  body state : Inport
  throttle : Inport  Port=2
  status : Inport  Port=3
  Bias : Bias  Bias=demo(3).torque_bias  SaturateOnIntegerOverflow=off
  Bus Selector : BusSelector  OutputSignals=groundspeed
  Bus Selector1 : BusSelector  OutputSignals=gear
  Gain1 : Gain  Gain=demo(3).torque_gain
  Gain2 : Gain  Gain=-demo(3).torque_rate
  Product : Product
  Saturation : Saturate  UpperLimit=inf  LowerLimit=0
  Saturation Dynamic2 : simulink/Discontinuities/Saturation Dynamic  OutMin=[]  OutMax=[]  OutDataTypeStr=Inherit: Same as second input  OutDataType=fixdt(1, 16)  OutScaling=2^-10  DoSatur=off
  Sign : Signum
  Zero : Constant  Value=0  OutDataTypeStr=Inherit: Inherit via back propagation
  total torque : Outport
  wires:
  Gain2/1 -> Bias/1
  Bias/1 -> Saturation/1
  Bus Selector/1 -> Gain2/1  "<groundspeed>"
  throttle/1 -> Gain1/1
  Saturation Dynamic2/1 -> Product/1
  Saturation/1 -> Saturation Dynamic2/1
  Sign/1 -> Product/2
  Zero/1 -> Saturation Dynamic2/3
  Product/1 -> total torque/1
  body state/1 -> Bus Selector/1
  status/1 -> Bus Selector1/1
  Gain1/1 -> Saturation Dynamic2/2
  Bus Selector1/1 -> Sign/1  "<gear>"

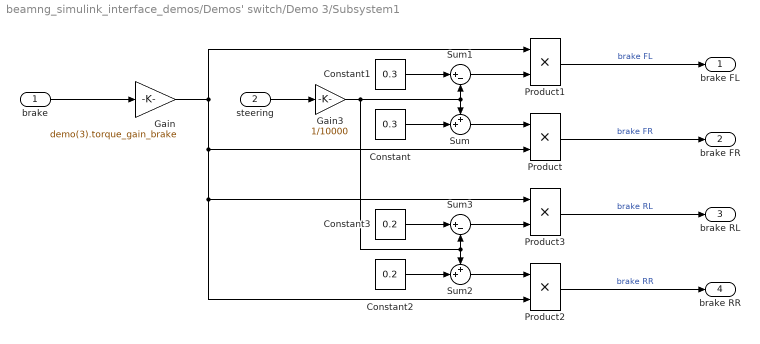
== system beamng_simulink_interface_demos/Demos' switch/Demo 3/Subsystem1 ==
  brake : Inport
  steering : Inport  Port=2
  Constant : Constant  Value=0.3
  Constant1 : Constant  Value=0.3
  Constant2 : Constant  Value=0.2
  Constant3 : Constant  Value=0.2
  Gain : Gain  Gain=demo(3).torque_gain_brake
  Gain3 : Gain  Gain=1/10000
  Product{,1..3} (4 alike) : Product
  Sum : Sum  Inputs=++|
  Sum1 : Sum  Inputs=|+-
  Sum2 : Sum  Inputs=++|
  Sum3 : Sum  Inputs=|+-
  brake FL : Outport
  brake FR : Outport  Port=2
  brake RL : Outport  Port=3
  brake RR : Outport  Port=4
  wires:
  brake/1 -> Gain/1
  Product/1 -> brake FR/1  "brake FR"
  Product3/1 -> brake RL/1  "brake RL"
  Product2/1 -> brake RR/1  "brake RR"
  Product1/1 -> brake FL/1  "brake FL"
  steering/1 -> Gain3/1
  Constant/1 -> Sum/2
  Sum/1 -> Product/1
  Sum1/1 -> Product1/2
  Constant1/1 -> Sum1/1
  Gain/1 -> Product1/1, Product2/2, Product3/1, Product/2
  Constant2/1 -> Sum2/2
  Gain3/1 -> Sum2/1, Sum3/2, Sum/1, Sum1/2
  Sum2/1 -> Product2/1
  Sum3/1 -> Product3/2
  Constant3/1 -> Sum3/1

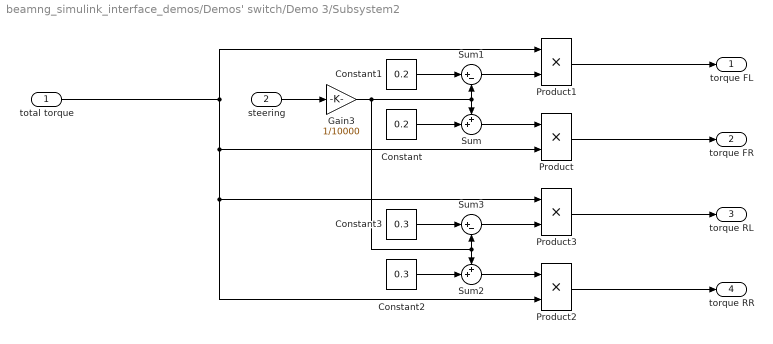
== system beamng_simulink_interface_demos/Demos' switch/Demo 3/Subsystem2 ==
  total torque : Inport
  steering : Inport  Port=2
  Constant : Constant  Value=0.2
  Constant1 : Constant  Value=0.2
  Constant2 : Constant  Value=0.3
  Constant3 : Constant  Value=0.3
  Gain3 : Gain  Gain=1/10000
  Product{,1..3} (4 alike) : Product
  Sum : Sum  Inputs=++|
  Sum1 : Sum  Inputs=|+-
  Sum2 : Sum  Inputs=++|
  Sum3 : Sum  Inputs=|+-
  torque FL : Outport
  torque FR : Outport  Port=2
  torque RL : Outport  Port=3
  torque RR : Outport  Port=4
  wires:
  Constant3/1 -> Sum3/1
  Sum3/1 -> Product3/2
  Sum2/1 -> Product2/1
  Gain3/1 -> Sum1/2, Sum/1, Sum3/2, Sum2/1
  Constant2/1 -> Sum2/2
  total torque/1 -> Product/2, Product3/1, Product2/2, Product1/1
  Constant1/1 -> Sum1/1
  Sum1/1 -> Product1/2
  Sum/1 -> Product/1
  Constant/1 -> Sum/2
  steering/1 -> Gain3/1
  Product1/1 -> torque FL/1
  Product2/1 -> torque RR/1
  Product3/1 -> torque RL/1
  Product/1 -> torque FR/1
